simulink model "GSM_sim_ISI"  (R2013a)
settings: Solver=VariableStepDiscrete  StartTime=0.0  StopTime=simulationTime  RelTol=1e-3
values from neighbouring files (symbols this model uses):
  lengthOfSymbol = 64    [M_PSK_config.m]    (also in modulationen_config.m)
  sampleTime = 1    [M_PSK_config.m]    (also in modulationen_config.m)
undefined symbols (not defined in the file or in its folder): rcRoll, rcUpsample
libraries: commchan3 x4, commfilt2 x3, commdigbbndpm3 x2, commdigbbndcpm2 x2, simulink x1, commutil2 x1, dspsigops x1
settings Model: Creator=Philipp Fetzer  LastModifiedBy=mainster
settings DataIOCC: SignalLoggingSaveFormat=ModelDataLogs
settings OptimizationCC: ExpressionDepthLimit=2147483647
settings DebuggingCC: FcnCallInpInsideContextMsg=UseLocalSettings  StrictBusMsg=Warning
settings GRTTargetCC: CombineOutputUpdateFcns=off  GRTInterface=on

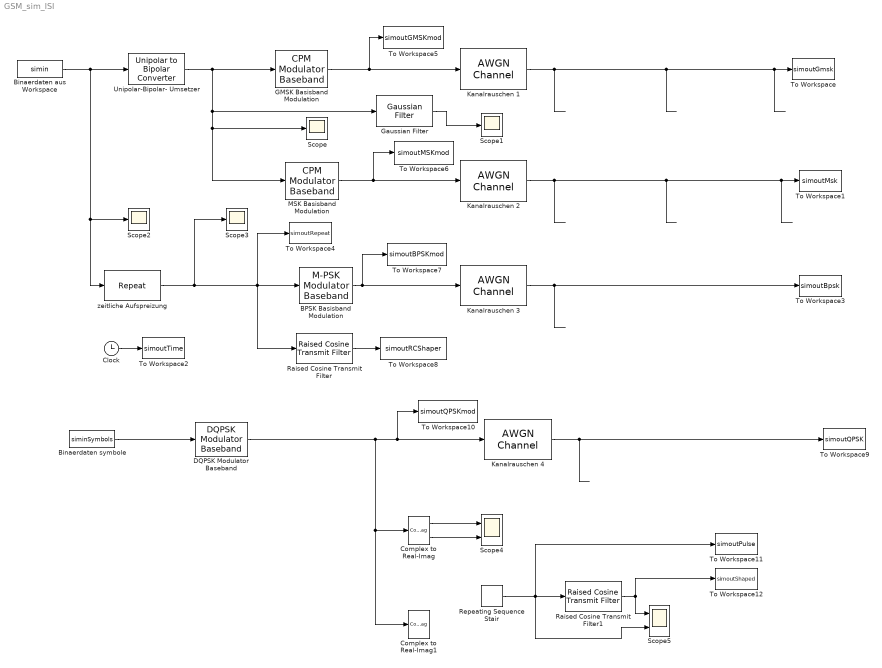
== system GSM_sim_ISI ==
  BPSK Basisband Modulation : commdigbbndpm3/M-PSK Modulator Baseband  M=2  InType=Integer  Enc=Binary  Mapping=[0:2]  Ph=phaseOffset  outDtype=double  outWordLen=16  outUDDataType=sfix(16)  outFracLenMode=Best precision  outFracLen=15
  Binaerdaten aus Workspace : FromWorkspace  VariableName=simin  SampleTime=sampleTime
  Binaerdaten symbole : FromWorkspace  VariableName=siminSymbols  SampleTime=sampleTime
  Clock : Clock
  Complex to Real-Imag : ComplexToRealImag
  Complex to Real-Imag1 : ComplexToRealImag
  DQPSK Modulator Baseband : commdigbbndpm3/DQPSK Modulator Baseband  InType=Integer  Enc=Gray  Ph=pi/4  outDtype=double
  GMSK Basisband Modulation : commdigbbndcpm2/CPM Modulator Baseband  Mnum=2  inputType=Integer  mappingType=Binary  modIdx=.5  pulseShape=Gaussian  BT=.3  mainLobePulseLength=0.2  rollOff=0.2  pulseLength=4  preHistory=1  phaseOffset=phaseOffset  samplesPerSymbol=lengthOfSymbol  RateOptions=Inherit from input (this choice will be removed - see release notes)  outDataType=double
  Gaussian Filter : commfilt2/Gaussian Filter  N=4  BT=0.3  D=2  sampMode=Frame-based  normMode=Sum of coefficients  filterGain=1  checkCoeff=off  variableName=gaussFilt  launchFVT=off  roundingMode=Floor  overflowMode=off  InputProcessing=Columns as channels (frame based)
  Kanalrauschen {1..4} (4 alike) : commchan3/AWGN Channel  InputProcessing=Inherited (this choice will be removed - see release notes)  seed=67  noiseMode="Signal to noise ratio  (SNR)"  EbNodB=30  EsNodB=10  SNRdB=SNR  bitsPerSym=1  Ps=1  Tsym=1  variance=1
  MSK Basisband Modulation : commdigbbndcpm2/CPM Modulator Baseband  Mnum=2  inputType=Integer  mappingType=Binary  modIdx=0.5  pulseShape=Rectangular  BT=0.3  mainLobePulseLength=0.2  rollOff=0.2  pulseLength=1  preHistory=1  phaseOffset=phaseOffset  samplesPerSymbol=lengthOfSymbol  RateOptions=Inherit from input (this choice will be removed - see release notes)  outDataType=double
  Raised Cosine Transmit Filter : commfilt2/Raised Cosine Transmit Filter  filtType=Normal  D=5  R=0.8  sampMode=Mute  saveAsFlag=0  N=8  framing=Enforce single-rate processing  InputProcessing=Columns as channels (frame based)  checkGain=Normalized  filterGain=1  checkCoeff=off  variableName=rcTxFilt  launchFVT=off  roundingMode=Floor  overflowMode=off
  Raised Cosine Transmit Filter1 : commfilt2/Raised Cosine Transmit Filter  filtType=Normal  D=10  R=rcRoll  sampMode=Mute  saveAsFlag=0  N=rcUpsample  framing=Allow multirate processing  checkGain=Normalized  filterGain=1  checkCoeff=on  variableName=rcTxFilt1  launchFVT=off  roundingMode=Floor  overflowMode=off
  Repeating Sequence Stair : simulink/Sources/Repeating Sequence Stair  OutValues=[0 0 1 0 0 0 0 0 0 0 0].'  tsamp=sampleTime  OutMin=[]  OutMax=[]  OutDataTypeStr=double  OutputDataTypeScalingMode=double  OutDataType=fixdt(0,8)  ConRadixGroup=Best Precision: Vector-wise  OutScaling=2^-12
  Scope{,1..3} (4 alike) : Scope
      Scope2 settings: SaveName=ScopeData2  MaxDataPoints=500000
      Scope3 settings: YMin=-2  YMax=2  SaveName=ScopeData3  MaxDataPoints=500000
  Scope4 : Scope  NumInputPorts=2
      settings: ShowLegends=on  TimeRange=14  YMin=-1~-1  YMax=1~1  SaveName=ScopeData4  MaxDataPoints=500000
  Scope5 : Scope  NumInputPorts=2
      settings: ShowLegends=on  TimeRange=14  YMin=-1.5~-1.5  YMax=1.5~1.5  SaveName=ScopeData5  MaxDataPoints=500000
  To Workspace : ToWorkspace  VariableName=simoutGmsk  SampleTime=-1  SaveFormat=Structure
  To Workspace1 : ToWorkspace  VariableName=simoutMsk  SampleTime=-1  SaveFormat=Structure
  To Workspace10 : ToWorkspace  VariableName=simoutQPSKmod  SampleTime=-1  SaveFormat=Structure
  To Workspace11 : ToWorkspace  VariableName=simoutPulse  SampleTime=-1  SaveFormat=Structure
  To Workspace12 : ToWorkspace  VariableName=simoutShaped  SampleTime=-1  SaveFormat=Structure
  To Workspace2 : ToWorkspace  VariableName=simoutTime  SampleTime=-1  SaveFormat=Structure
  To Workspace3 : ToWorkspace  VariableName=simoutBpsk  SampleTime=-1  SaveFormat=Structure
  To Workspace4 : ToWorkspace  VariableName=simoutRepeat  SampleTime=-1  SaveFormat=Structure
  To Workspace5 : ToWorkspace  VariableName=simoutGMSKmod  SampleTime=-1  SaveFormat=Structure
  To Workspace6 : ToWorkspace  VariableName=simoutMSKmod  SampleTime=-1  SaveFormat=Structure
  To Workspace7 : ToWorkspace  VariableName=simoutBPSKmod  SampleTime=-1  SaveFormat=Structure
  To Workspace8 : ToWorkspace  VariableName=simoutRCShaper  SampleTime=-1  SaveFormat=Structure
  To Workspace9 : ToWorkspace  VariableName=simoutQPSK  SampleTime=-1  SaveFormat=Structure
  Unipolar-Bipolar- Umsetzer : commutil2/Unipolar to Bipolar Converter  M=2  polarity=Positive  dataType=Inherit via internal rule
  zeitliche Aufspreizung : dspsigops/Repeat  N=lengthOfSymbol  InputProcessing=Inherited (this choice will be removed - see release notes)  RateOptions=Allow multirate processing  ic=0  mode=Unused parameter value
  wires:
  Unipolar-Bipolar- Umsetzer/1 -> GMSK Basisband Modulation/1, Scope/1, MSK Basisband Modulation/1, Gaussian Filter/1
  MSK Basisband Modulation/1 -> Kanalrauschen 2/1, To Workspace6/1
  Binaerdaten aus Workspace/1 -> Unipolar-Bipolar- Umsetzer/1, Scope2/1, zeitliche Aufspreizung/1
  Clock/1 -> To Workspace2/1
  Kanalrauschen 1/1 -> To Workspace/1
  GMSK Basisband Modulation/1 -> Kanalrauschen 1/1, To Workspace5/1
  BPSK Basisband Modulation/1 -> Kanalrauschen 3/1, To Workspace7/1
  Kanalrauschen 2/1 -> To Workspace1/1
  Kanalrauschen 3/1 -> To Workspace3/1
  Gaussian Filter/1 -> Scope1/1
  Raised Cosine Transmit Filter/1 -> To Workspace8/1
  Kanalrauschen 4/1 -> To Workspace9/1
  Binaerdaten symbole/1 -> DQPSK Modulator Baseband/1
  zeitliche Aufspreizung/1 -> Scope3/1, To Workspace4/1, BPSK Basisband Modulation/1, Raised Cosine Transmit Filter/1
  Complex to Real-Imag/1 -> Scope4/1
  Complex to Real-Imag/2 -> Scope4/2
  Raised Cosine Transmit Filter1/1 -> To Workspace12/1, Scope5/1
  Repeating Sequence Stair/1 -> Raised Cosine Transmit Filter1/1, To Workspace11/1, Scope5/2
  DQPSK Modulator Baseband/1 -> Complex to Real-Imag1/1, Complex to Real-Imag/1, Kanalrauschen 4/1, To Workspace10/1
